simulink library "Encoders_Lib"  (Simulink 8.7)
settings: Solver=ode45  StartTime=0.0  StopTime=10.0  RelTol=1e-3
settings Model: Creator=uzivatel  LastModifiedBy=Jozko Mrkvicka

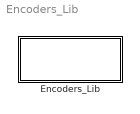
== system Encoders_Lib ==
  Encoders_Lib : Subsystem

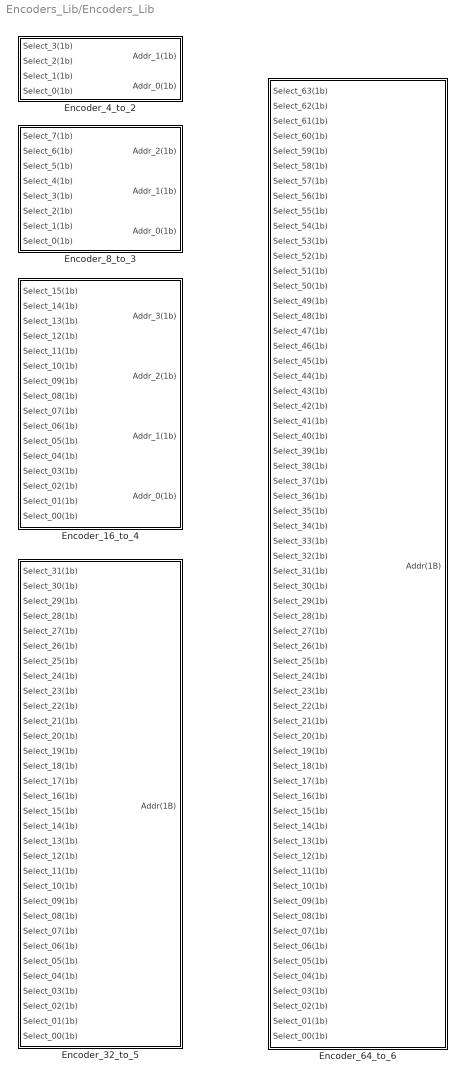
== system Encoders_Lib/Encoders_Lib ==
  Encoder_16_to_4 : Subsystem
  Encoder_32_to_5 : Subsystem
  Encoder_4_to_2 : Subsystem
  Encoder_64_to_6 : Subsystem
  Encoder_8_to_3 : Subsystem

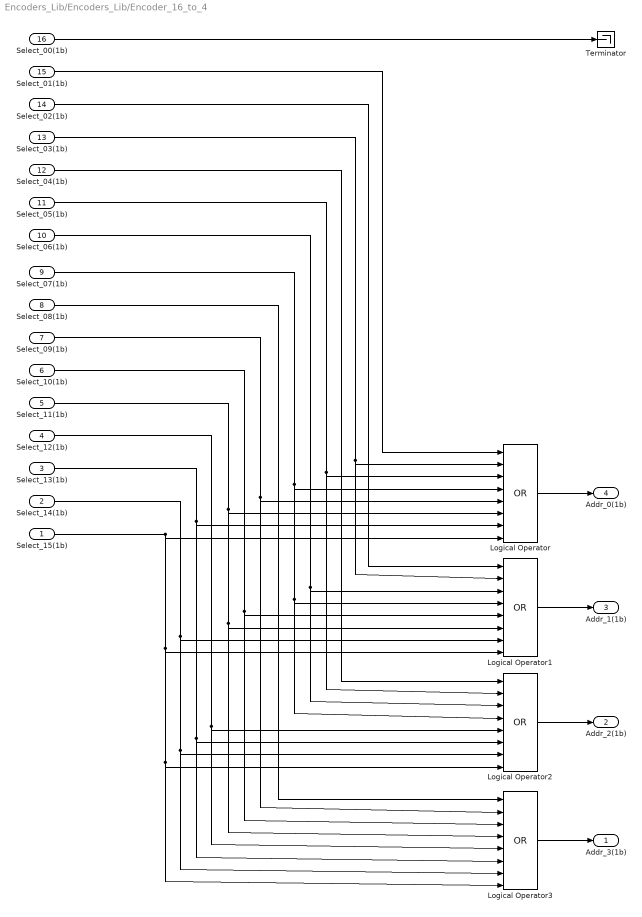
== system Encoders_Lib/Encoders_Lib/Encoder_16_to_4 ==
  Select_15(1b) : Inport
  Select_14(1b) : Inport  Port=2
  Select_13(1b) : Inport  Port=3
  Select_12(1b) : Inport  Port=4
  Select_11(1b) : Inport  Port=5
  Select_10(1b) : Inport  Port=6
  Select_09(1b) : Inport  Port=7
  Select_08(1b) : Inport  Port=8
  Select_07(1b) : Inport  Port=9
  Select_06(1b) : Inport  Port=10
  Select_05(1b) : Inport  Port=11
  Select_04(1b) : Inport  Port=12
  Select_03(1b) : Inport  Port=13
  Select_02(1b) : Inport  Port=14
  "Select_01(1b) " : Inport  Port=15
  Select_00(1b) : Inport  Port=16
  Logical Operator{,1..3} (4 alike) : Logic  Operator=OR  Inputs=8  IconShape=distinctive  AllPortsSameDT=off  OutDataTypeStr=boolean
  Terminator : Terminator
  Addr_3(1b) : Outport
  Addr_2(1b) : Outport  Port=2
  Addr_1(1b) : Outport  Port=3
  Addr_0(1b) : Outport  Port=4
  wires:
  Logical Operator/1 -> Addr_0(1b)/1
  Logical Operator1/1 -> Addr_1(1b)/1
  Logical Operator2/1 -> Addr_2(1b)/1
  Logical Operator3/1 -> Addr_3(1b)/1
  "Select_01(1b) "/1 -> Logical Operator/1
  Select_02(1b)/1 -> Logical Operator1/1
  Select_03(1b)/1 -> Logical Operator1/2, Logical Operator/2
  Select_04(1b)/1 -> Logical Operator2/1
  Select_05(1b)/1 -> Logical Operator2/2, Logical Operator/3
  Select_06(1b)/1 -> Logical Operator2/3, Logical Operator1/3
  Select_07(1b)/1 -> Logical Operator2/4, Logical Operator1/4, Logical Operator/4
  Select_08(1b)/1 -> Logical Operator3/1
  Select_09(1b)/1 -> Logical Operator3/2, Logical Operator/5
  Select_10(1b)/1 -> Logical Operator3/3, Logical Operator1/5
  Select_11(1b)/1 -> Logical Operator3/4, Logical Operator1/6, Logical Operator/6
  Select_12(1b)/1 -> Logical Operator3/5, Logical Operator2/5
  Select_13(1b)/1 -> Logical Operator3/6, Logical Operator2/6, Logical Operator/7
  Select_14(1b)/1 -> Logical Operator3/7, Logical Operator2/7, Logical Operator1/7
  Select_15(1b)/1 -> Logical Operator3/8, Logical Operator2/8, Logical Operator1/8, Logical Operator/8
  Select_00(1b)/1 -> Terminator/1

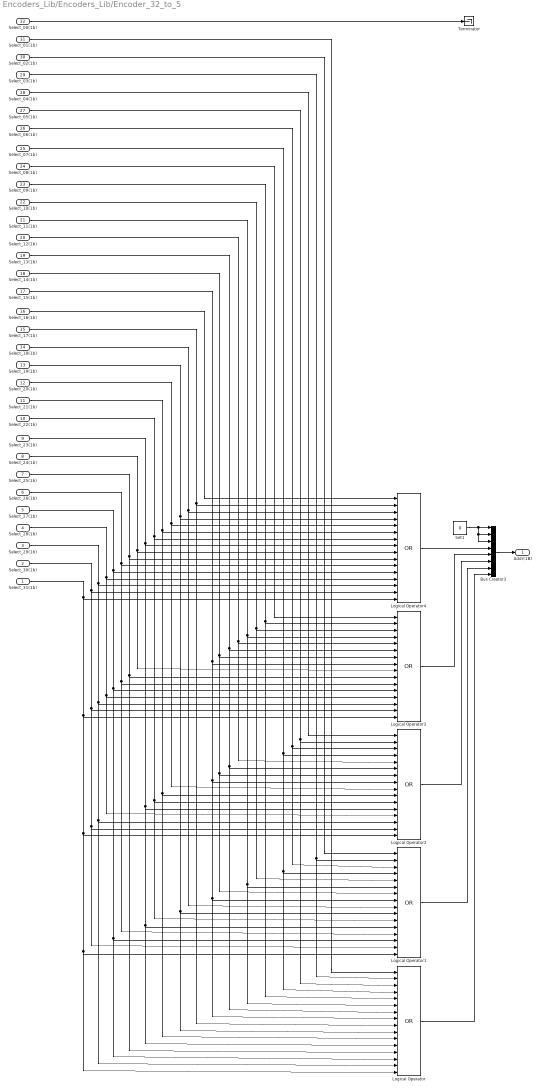
== system Encoders_Lib/Encoders_Lib/Encoder_32_to_5 ==
  Select_31(1b) : Inport
  Select_30(1b) : Inport  Port=2
  Select_29(1b) : Inport  Port=3
  Select_28(1b) : Inport  Port=4
  Select_27(1b) : Inport  Port=5
  Select_26(1b) : Inport  Port=6
  Select_25(1b) : Inport  Port=7
  Select_24(1b) : Inport  Port=8
  Select_23(1b) : Inport  Port=9
  Select_22(1b) : Inport  Port=10
  Select_21(1b) : Inport  Port=11
  Select_20(1b) : Inport  Port=12
  Select_19(1b) : Inport  Port=13
  Select_18(1b) : Inport  Port=14
  Select_17(1b) : Inport  Port=15
  Select_16(1b) : Inport  Port=16
  Select_15(1b) : Inport  Port=17
  Select_14(1b) : Inport  Port=18
  Select_13(1b) : Inport  Port=19
  Select_12(1b) : Inport  Port=20
  Select_11(1b) : Inport  Port=21
  Select_10(1b) : Inport  Port=22
  Select_09(1b) : Inport  Port=23
  Select_08(1b) : Inport  Port=24
  Select_07(1b) : Inport  Port=25
  Select_06(1b) : Inport  Port=26
  Select_05(1b) : Inport  Port=27
  Select_04(1b) : Inport  Port=28
  Select_03(1b) : Inport  Port=29
  Select_02(1b) : Inport  Port=30
  "Select_01(1b) " : Inport  Port=31
  Select_00(1b) : Inport  Port=32
  Bus Creator3 : BusCreator  Inputs=8
  Logical Operator{,1..4} (5 alike) : Logic  Operator=OR  Inputs=16  IconShape=distinctive  AllPortsSameDT=off  OutDataTypeStr=boolean
  Set1 : Constant  Value=0  OutDataTypeStr=boolean
  Terminator : Terminator
  Addr(1B) : Outport
  wires:
  Bus Creator3/1 -> Addr(1B)/1
  Set1/1 -> Bus Creator3/2, Bus Creator3/3, Bus Creator3/1
  Logical Operator/1 -> Bus Creator3/8
  Logical Operator1/1 -> Bus Creator3/7
  Logical Operator2/1 -> Bus Creator3/6
  Logical Operator3/1 -> Bus Creator3/5
  "Select_01(1b) "/1 -> Logical Operator/1
  Select_02(1b)/1 -> Logical Operator1/1
  Select_03(1b)/1 -> Logical Operator1/2, Logical Operator/2
  Select_04(1b)/1 -> Logical Operator2/1
  Select_05(1b)/1 -> Logical Operator2/2, Logical Operator/3
  Select_06(1b)/1 -> Logical Operator2/3, Logical Operator1/3
  Select_07(1b)/1 -> Logical Operator2/4, Logical Operator1/4, Logical Operator/4
  Select_08(1b)/1 -> Logical Operator3/1
  Select_09(1b)/1 -> Logical Operator3/2, Logical Operator/5
  Select_10(1b)/1 -> Logical Operator3/3, Logical Operator1/5
  Select_11(1b)/1 -> Logical Operator3/4, Logical Operator1/6, Logical Operator/6
  Select_12(1b)/1 -> Logical Operator3/5, Logical Operator2/5
  Select_13(1b)/1 -> Logical Operator3/6, Logical Operator2/6, Logical Operator/7
  Select_14(1b)/1 -> Logical Operator3/7, Logical Operator2/7, Logical Operator1/7
  Select_15(1b)/1 -> Logical Operator3/8, Logical Operator2/8, Logical Operator1/8, Logical Operator/8
  Select_00(1b)/1 -> Terminator/1
  Logical Operator4/1 -> Bus Creator3/4
  Select_16(1b)/1 -> Logical Operator4/1
  Select_17(1b)/1 -> Logical Operator4/2, Logical Operator/9
  Select_18(1b)/1 -> Logical Operator4/3, Logical Operator1/9
  Select_19(1b)/1 -> Logical Operator4/4, Logical Operator1/10, Logical Operator/10
  Select_20(1b)/1 -> Logical Operator4/5, Logical Operator2/9
  Select_21(1b)/1 -> Logical Operator4/6, Logical Operator2/10, Logical Operator/11
  Select_22(1b)/1 -> Logical Operator4/7, Logical Operator2/11, Logical Operator1/11
  Select_23(1b)/1 -> Logical Operator4/8, Logical Operator2/12, Logical Operator1/12, Logical Operator/12
  Select_24(1b)/1 -> Logical Operator4/9, Logical Operator3/9
  Select_25(1b)/1 -> Logical Operator4/10, Logical Operator3/10, Logical Operator/13
  Select_26(1b)/1 -> Logical Operator4/11, Logical Operator3/11, Logical Operator1/13
  Select_27(1b)/1 -> Logical Operator4/12, Logical Operator3/12, Logical Operator1/14, Logical Operator/14
  Select_28(1b)/1 -> Logical Operator4/13, Logical Operator3/13, Logical Operator2/13
  Select_29(1b)/1 -> Logical Operator4/14, Logical Operator3/14, Logical Operator2/14, Logical Operator/15
  Select_30(1b)/1 -> Logical Operator4/15, Logical Operator3/15, Logical Operator2/15, Logical Operator1/15
  Select_31(1b)/1 -> Logical Operator4/16, Logical Operator3/16, Logical Operator2/16, Logical Operator1/16, Logical Operator/16

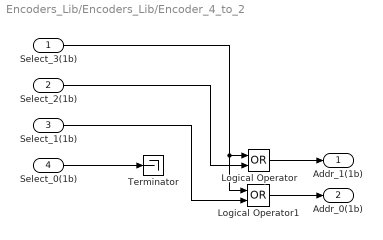
== system Encoders_Lib/Encoders_Lib/Encoder_4_to_2 ==
  Select_3(1b) : Inport
  "Select_2(1b) " : Inport  Port=2
  Select_1(1b) : Inport  Port=3
  Select_0(1b) : Inport  Port=4
  Logical Operator : Logic  Operator=OR  IconShape=distinctive  AllPortsSameDT=off  OutDataTypeStr=boolean
  Logical Operator1 : Logic  Operator=OR  IconShape=distinctive  AllPortsSameDT=off  OutDataTypeStr=boolean
  Terminator : Terminator
  Addr_1(1b) : Outport
  Addr_0(1b) : Outport  Port=2
  wires:
  Logical Operator/1 -> Addr_1(1b)/1
  Logical Operator1/1 -> Addr_0(1b)/1
  "Select_2(1b) "/1 -> Logical Operator/2
  Select_1(1b)/1 -> Logical Operator1/2
  Select_0(1b)/1 -> Terminator/1
  Select_3(1b)/1 -> Logical Operator/1, Logical Operator1/1

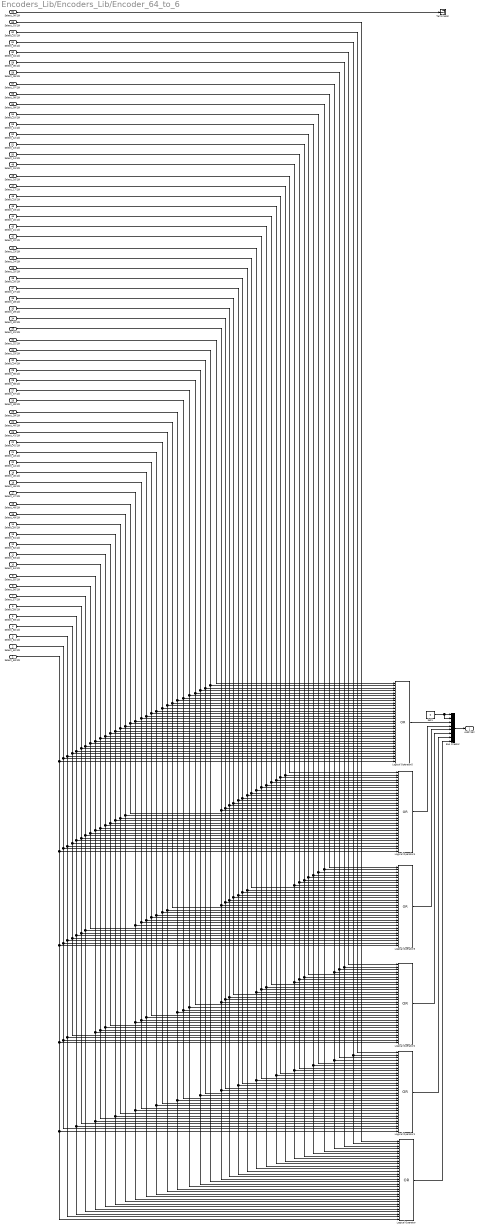
== system Encoders_Lib/Encoders_Lib/Encoder_64_to_6 ==
  Select_63(1b) : Inport
  Select_62(1b) : Inport  Port=2
  Select_61(1b) : Inport  Port=3
  Select_60(1b) : Inport  Port=4
  Select_59(1b) : Inport  Port=5
  Select_58(1b) : Inport  Port=6
  Select_57(1b) : Inport  Port=7
  Select_56(1b) : Inport  Port=8
  Select_55(1b) : Inport  Port=9
  Select_54(1b) : Inport  Port=10
  Select_53(1b) : Inport  Port=11
  Select_52(1b) : Inport  Port=12
  Select_51(1b) : Inport  Port=13
  Select_50(1b) : Inport  Port=14
  Select_49(1b) : Inport  Port=15
  Select_48(1b) : Inport  Port=16
  Select_47(1b) : Inport  Port=17
  Select_46(1b) : Inport  Port=18
  Select_45(1b) : Inport  Port=19
  Select_44(1b) : Inport  Port=20
  Select_43(1b) : Inport  Port=21
  Select_42(1b) : Inport  Port=22
  Select_41(1b) : Inport  Port=23
  Select_40(1b) : Inport  Port=24
  Select_39(1b) : Inport  Port=25
  Select_38(1b) : Inport  Port=26
  Select_37(1b) : Inport  Port=27
  Select_36(1b) : Inport  Port=28
  Select_35(1b) : Inport  Port=29
  Select_34(1b) : Inport  Port=30
  Select_33(1b) : Inport  Port=31
  Select_32(1b) : Inport  Port=32
  Select_31(1b) : Inport  Port=33
  Select_30(1b) : Inport  Port=34
  Select_29(1b) : Inport  Port=35
  Select_28(1b) : Inport  Port=36
  Select_27(1b) : Inport  Port=37
  Select_26(1b) : Inport  Port=38
  Select_25(1b) : Inport  Port=39
  Select_24(1b) : Inport  Port=40
  Select_23(1b) : Inport  Port=41
  Select_22(1b) : Inport  Port=42
  Select_21(1b) : Inport  Port=43
  Select_20(1b) : Inport  Port=44
  Select_19(1b) : Inport  Port=45
  Select_18(1b) : Inport  Port=46
  Select_17(1b) : Inport  Port=47
  Select_16(1b) : Inport  Port=48
  Select_15(1b) : Inport  Port=49
  Select_14(1b) : Inport  Port=50
  Select_13(1b) : Inport  Port=51
  Select_12(1b) : Inport  Port=52
  Select_11(1b) : Inport  Port=53
  Select_10(1b) : Inport  Port=54
  Select_09(1b) : Inport  Port=55
  Select_08(1b) : Inport  Port=56
  Select_07(1b) : Inport  Port=57
  Select_06(1b) : Inport  Port=58
  Select_05(1b) : Inport  Port=59
  Select_04(1b) : Inport  Port=60
  Select_03(1b) : Inport  Port=61
  Select_02(1b) : Inport  Port=62
  "Select_01(1b) " : Inport  Port=63
  Select_00(1b) : Inport  Port=64
  Bus Creator : BusCreator  Inputs=8
  Logical Operator{,1..5} (6 alike) : Logic  Operator=OR  Inputs=32  IconShape=distinctive  AllPortsSameDT=off  OutDataTypeStr=boolean
  Set1 : Constant  Value=0  OutDataTypeStr=boolean
  Terminator : Terminator
  Addr(1B) : Outport
  wires:
  Bus Creator/1 -> Addr(1B)/1
  Set1/1 -> Bus Creator/2, Bus Creator/1
  Logical Operator/1 -> Bus Creator/8
  Logical Operator1/1 -> Bus Creator/7
  Logical Operator2/1 -> Bus Creator/6
  Logical Operator3/1 -> Bus Creator/5
  "Select_01(1b) "/1 -> Logical Operator/1
  Select_02(1b)/1 -> Logical Operator1/1
  Select_03(1b)/1 -> Logical Operator/2, Logical Operator1/2
  Select_04(1b)/1 -> Logical Operator2/1
  Select_05(1b)/1 -> Logical Operator/3, Logical Operator2/2
  Select_06(1b)/1 -> Logical Operator1/3, Logical Operator2/3
  Select_07(1b)/1 -> Logical Operator/4, Logical Operator1/4, Logical Operator2/4
  Select_08(1b)/1 -> Logical Operator3/1
  Select_09(1b)/1 -> Logical Operator/5, Logical Operator3/2
  Select_10(1b)/1 -> Logical Operator1/5, Logical Operator3/3
  Select_11(1b)/1 -> Logical Operator/6, Logical Operator1/6, Logical Operator3/4
  Select_12(1b)/1 -> Logical Operator2/5, Logical Operator3/5
  Select_13(1b)/1 -> Logical Operator/7, Logical Operator2/6, Logical Operator3/6
  Select_14(1b)/1 -> Logical Operator3/7, Logical Operator1/7, Logical Operator2/7
  Select_15(1b)/1 -> Logical Operator/8, Logical Operator1/8, Logical Operator2/8, Logical Operator3/8
  Select_00(1b)/1 -> Terminator/1
  Logical Operator4/1 -> Bus Creator/4
  Select_16(1b)/1 -> Logical Operator4/1
  Select_17(1b)/1 -> Logical Operator/9, Logical Operator4/2
  Select_18(1b)/1 -> Logical Operator1/9, Logical Operator4/3
  Select_19(1b)/1 -> Logical Operator/10, Logical Operator1/10, Logical Operator4/4
  Select_20(1b)/1 -> Logical Operator2/9, Logical Operator4/5
  Select_21(1b)/1 -> Logical Operator/11, Logical Operator2/10, Logical Operator4/6
  Select_22(1b)/1 -> Logical Operator1/11, Logical Operator2/11, Logical Operator4/7
  Select_23(1b)/1 -> Logical Operator/12, Logical Operator1/12, Logical Operator2/12, Logical Operator4/8
  Select_24(1b)/1 -> Logical Operator3/9, Logical Operator4/9
  Select_25(1b)/1 -> Logical Operator/13, Logical Operator3/10, Logical Operator4/10
  Select_26(1b)/1 -> Logical Operator1/13, Logical Operator3/11, Logical Operator4/11
  Select_27(1b)/1 -> Logical Operator/14, Logical Operator1/14, Logical Operator3/12, Logical Operator4/12
  Select_28(1b)/1 -> Logical Operator2/13, Logical Operator3/13, Logical Operator4/13
  Select_29(1b)/1 -> Logical Operator/15, Logical Operator2/14, Logical Operator3/14, Logical Operator4/14
  Select_30(1b)/1 -> Logical Operator1/15, Logical Operator2/15, Logical Operator3/15, Logical Operator4/15
  Select_31(1b)/1 -> Logical Operator/16, Logical Operator1/16, Logical Operator2/16, Logical Operator3/16, Logical Operator4/16
  Logical Operator5/1 -> Bus Creator/3
  Select_32(1b)/1 -> Logical Operator5/1
  Select_33(1b)/1 -> Logical Operator/17, Logical Operator5/2
  Select_34(1b)/1 -> Logical Operator1/17, Logical Operator5/3
  Select_35(1b)/1 -> Logical Operator/18, Logical Operator1/18, Logical Operator5/4
  Select_36(1b)/1 -> Logical Operator2/17, Logical Operator5/5
  Select_37(1b)/1 -> Logical Operator2/18, Logical Operator/19, Logical Operator5/6
  Select_39(1b)/1 -> Logical Operator1/20, Logical Operator/20, Logical Operator2/20, Logical Operator5/8
  Select_38(1b)/1 -> Logical Operator1/19, Logical Operator2/19, Logical Operator5/7
  Select_40(1b)/1 -> Logical Operator3/17, Logical Operator5/9
  Select_41(1b)/1 -> Logical Operator/21, Logical Operator3/18, Logical Operator5/10
  Select_43(1b)/1 -> Logical Operator3/20, Logical Operator/22, Logical Operator1/22, Logical Operator5/12
  Select_44(1b)/1 -> Logical Operator2/21, Logical Operator3/21, Logical Operator5/13
  Select_45(1b)/1 -> Logical Operator3/22, Logical Operator2/22, Logical Operator/23, Logical Operator5/14
  Select_46(1b)/1 -> Logical Operator1/23, Logical Operator2/23, Logical Operator3/23, Logical Operator5/15
  Select_47(1b)/1 -> Logical Operator3/24, Logical Operator1/24, Logical Operator/24, Logical Operator2/24, Logical Operator5/16
  Select_48(1b)/1 -> Logical Operator4/17, Logical Operator5/17
  Select_49(1b)/1 -> Logical Operator4/18, Logical Operator/25, Logical Operator5/18
  Select_50(1b)/1 -> Logical Operator1/25, Logical Operator4/19, Logical Operator5/19
  Select_51(1b)/1 -> Logical Operator1/26, Logical Operator/26, Logical Operator4/20, Logical Operator5/20
  Select_52(1b)/1 -> Logical Operator2/25, Logical Operator4/21, Logical Operator5/21
  Select_53(1b)/1 -> Logical Operator4/22, Logical Operator2/26, Logical Operator/27, Logical Operator5/22
  Select_55(1b)/1 -> Logical Operator4/24, Logical Operator2/28, Logical Operator1/28, Logical Operator/28, Logical Operator5/24
  Select_56(1b)/1 -> Logical Operator3/25, Logical Operator4/25, Logical Operator5/25
  Select_57(1b)/1 -> Logical Operator4/26, Logical Operator3/26, Logical Operator/29, Logical Operator5/26
  Select_58(1b)/1 -> Logical Operator1/29, Logical Operator3/27, Logical Operator4/27, Logical Operator5/27
  Select_59(1b)/1 -> Logical Operator3/28, Logical Operator/30, Logical Operator1/30, Logical Operator4/28, Logical Operator5/28
  Select_61(1b)/1 -> Logical Operator4/30, Logical Operator3/30, Logical Operator/31, Logical Operator2/30, Logical Operator5/30
  Select_62(1b)/1 -> Logical Operator1/31, Logical Operator2/31, Logical Operator3/31, Logical Operator4/31, Logical Operator5/31
  Select_63(1b)/1 -> Logical Operator3/32, Logical Operator1/32, Logical Operator/32, Logical Operator2/32, Logical Operator4/32, Logical Operator5/32
  Select_42(1b)/1 -> Logical Operator1/21, Logical Operator3/19, Logical Operator5/11
  Select_54(1b)/1 -> Logical Operator1/27, Logical Operator2/27, Logical Operator4/23, Logical Operator5/23
  Select_60(1b)/1 -> Logical Operator2/29, Logical Operator3/29, Logical Operator4/29, Logical Operator5/29

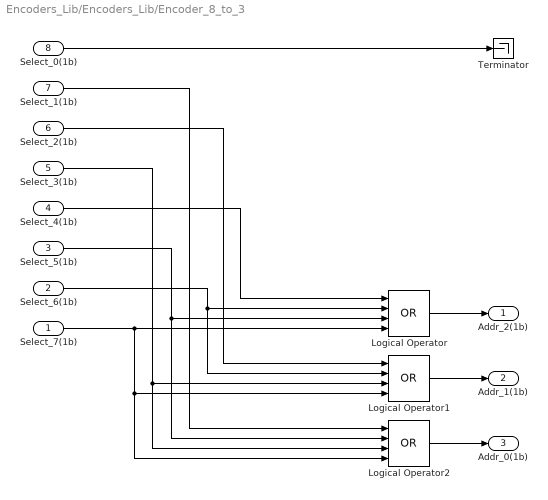
== system Encoders_Lib/Encoders_Lib/Encoder_8_to_3 ==
  Select_7(1b) : Inport
  Select_6(1b) : Inport  Port=2
  Select_5(1b) : Inport  Port=3
  "Select_4(1b) " : Inport  Port=4
  Select_3(1b) : Inport  Port=5
  Select_2(1b) : Inport  Port=6
  Select_1(1b) : Inport  Port=7
  Select_0(1b) : Inport  Port=8
  Logical Operator : Logic  Operator=OR  Inputs=4  IconShape=distinctive  AllPortsSameDT=off  OutDataTypeStr=boolean
  Logical Operator1 : Logic  Operator=OR  Inputs=4  IconShape=distinctive  AllPortsSameDT=off  OutDataTypeStr=boolean
  Logical Operator2 : Logic  Operator=OR  Inputs=4  IconShape=distinctive  AllPortsSameDT=off  OutDataTypeStr=boolean
  Terminator : Terminator
  Addr_2(1b) : Outport
  Addr_1(1b) : Outport  Port=2
  Addr_0(1b) : Outport  Port=3
  wires:
  Logical Operator/1 -> Addr_2(1b)/1
  Logical Operator1/1 -> Addr_1(1b)/1
  Logical Operator2/1 -> Addr_0(1b)/1
  "Select_4(1b) "/1 -> Logical Operator/1
  Select_2(1b)/1 -> Logical Operator1/1
  Select_6(1b)/1 -> Logical Operator1/2, Logical Operator/2
  Select_1(1b)/1 -> Logical Operator2/1
  Select_5(1b)/1 -> Logical Operator2/2, Logical Operator/3
  Select_3(1b)/1 -> Logical Operator2/3, Logical Operator1/3
  Select_7(1b)/1 -> Logical Operator2/4, Logical Operator1/4, Logical Operator/4
  Select_0(1b)/1 -> Terminator/1
